simulink model "joystick_mac_sub"  (Simulink 7.8)
settings: Solver=ode45  StartTime=0.0  StopTime=inf  RelTol=1e-3
values from neighbouring files (symbols this model uses):
  dt_sim = 0.005    [Init.m]
undefined symbols (not defined in the file or in its folder): waitfortreal
settings Model: Creator=sven  LastModifiedBy=sven

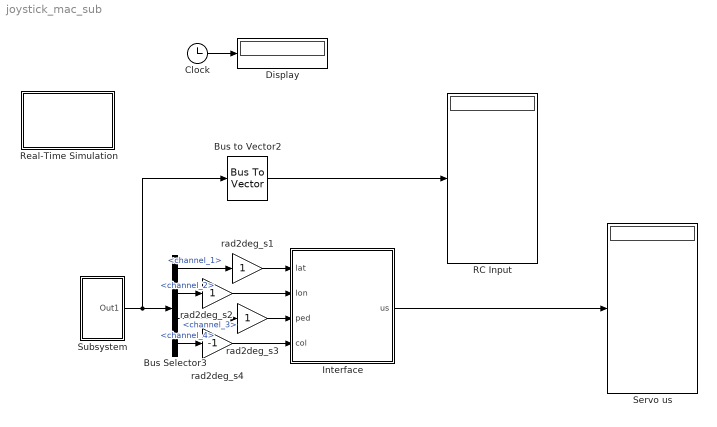
== system joystick_mac_sub ==
  Bus Selector3 : BusSelector  OutputSignals=channel_1,channel_2,channel_3,channel_4
  Bus to Vector2 : BusToVector
  Clock : Clock
  Display : Display
  Interface : Subsystem
  RC Input : Display
  Real-Time Simulation : Subsystem
      mask Display: disp('SL RT')
  Servo us : Display
  Subsystem : Subsystem
  rad2deg_s1 : Gain
  rad2deg_s2 : Gain
  rad2deg_s3 : Gain
  rad2deg_s4 : Gain  Gain=-1
  wires:
  Interface/1(us) -> Servo us/1
  Subsystem/1(Out1) -> Bus Selector3/1, Bus to Vector2/1
  Bus Selector3/1 -> rad2deg_s1/1  "<channel_1>"
  Bus Selector3/2 -> rad2deg_s2/1  "<channel_2>"
  Bus to Vector2/1 -> RC Input/1
  rad2deg_s1/1 -> Interface/1(lat)
  rad2deg_s2/1 -> Interface/2(lon)
  rad2deg_s3/1 -> Interface/3(ped)
  rad2deg_s4/1 -> Interface/4(col)
  Clock/1 -> Display/1
  Bus Selector3/3 -> rad2deg_s3/1  "<channel_3>"
  Bus Selector3/4 -> rad2deg_s4/1  "<channel_4>"

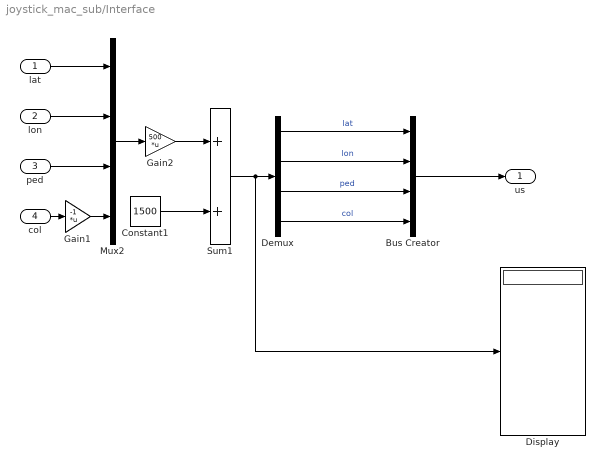
== system joystick_mac_sub/Interface ==
  lat : Inport
  lon : Inport  Port=2
  ped : Inport  Port=3
  col : Inport  Port=4
  Bus Creator : BusCreator
  Constant1 : Constant  Value=1500
  Demux : Demux
  Display : Display
  Gain1 : Gain  Gain=-1  Multiplication=Matrix(K*u)  SaturateOnIntegerOverflow=on  OutDataTypeStr=Inherit: Same as input  ParamDataTypeStr=Inherit: Same as input
  Gain2 : Gain  Gain=500  Multiplication=Matrix(K*u)  SaturateOnIntegerOverflow=on  OutDataTypeStr=Inherit: Same as input  ParamDataTypeStr=Inherit: Same as input
  Mux2 : Mux
  Sum1 : Sum  SaturateOnIntegerOverflow=on
  us : Outport
  wires:
  Mux2/1 -> Gain2/1
  lat/1 -> Mux2/1
  lon/1 -> Mux2/2
  ped/1 -> Mux2/3
  col/1 -> Gain1/1
  Constant1/1 -> Sum1/2
  Gain2/1 -> Sum1/1
  Gain1/1 -> Mux2/4
  Sum1/1 -> Demux/1, Display/1
  Demux/1 -> Bus Creator/1  "lat"
  Demux/2 -> Bus Creator/2  "lon"
  Demux/3 -> Bus Creator/3  "ped"
  Demux/4 -> Bus Creator/4  "col"
  Bus Creator/1 -> us/1

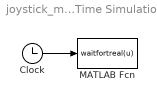
== system joystick_mac_sub/Real-Time Simulation ==
  Clock : Clock
  MATLAB Fcn : MATLABFcn  MATLABFcn=waitfortreal(u)  OutputDimensions=0
  wires:
  Clock/1 -> MATLAB Fcn/1

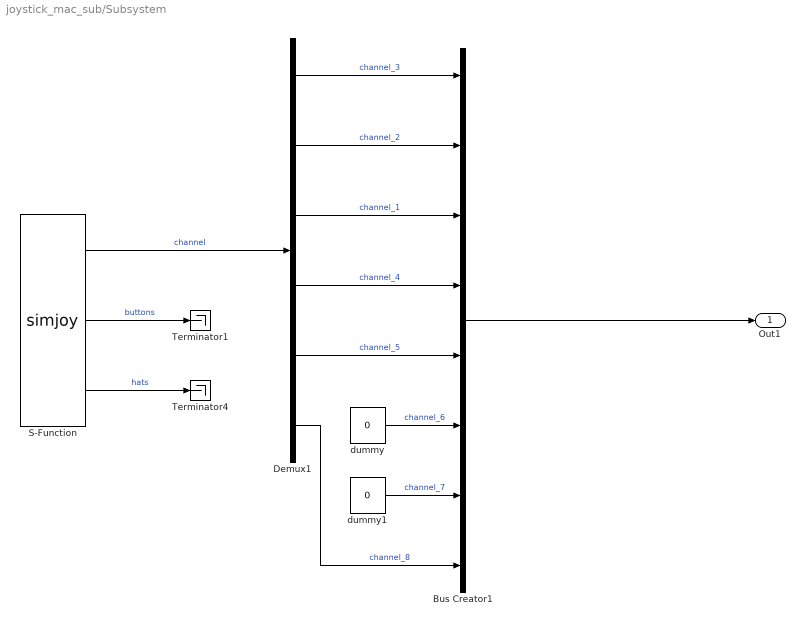
== system joystick_mac_sub/Subsystem ==
  Bus Creator1 : BusCreator  Inputs=8
  Demux1 : Demux  Outputs=6
  S-Function : S-Function  FunctionName=simjoy  Parameters=0  EnableBusSupport=off
  Terminator1 : Terminator
  Terminator4 : Terminator
  dummy : Constant  Value=0  SampleTime=dt_sim
  dummy1 : Constant  Value=0  SampleTime=dt_sim
  Out1 : Outport
  wires:
  dummy1/1 -> Bus Creator1/7  "channel_7"
  dummy/1 -> Bus Creator1/6  "channel_6"
  S-Function/1 -> Demux1/1  "channel"
  Demux1/1 -> Bus Creator1/1  "channel_3"
  Demux1/2 -> Bus Creator1/2  "channel_2"
  Demux1/3 -> Bus Creator1/3  "channel_1"
  Demux1/4 -> Bus Creator1/4  "channel_4"
  Demux1/5 -> Bus Creator1/5  "channel_5"
  Demux1/6 -> Bus Creator1/8  "channel_8"
  Bus Creator1/1 -> Out1/1
  S-Function/2 -> Terminator1/1  "buttons"
  S-Function/3 -> Terminator4/1  "hats"
